simulink model "demo_comp_imu"  (R2025a)
settings: Solver=VariableStepAuto  StartTime=0.0  StopTime=5  RelTol=1e-3
settings Model: Creator=xing2  LastModifiedBy=xing2

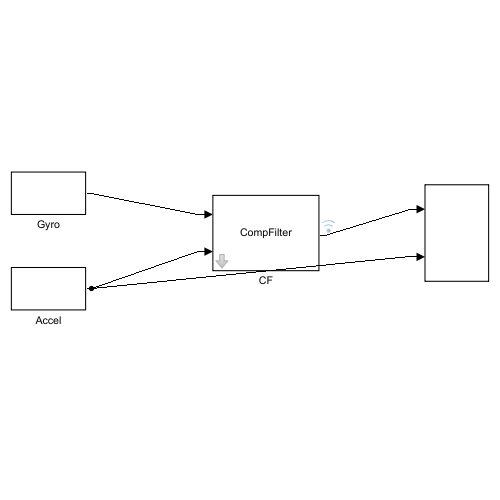
[thumbnail: Simulink's stored preview of the top-level diagram]
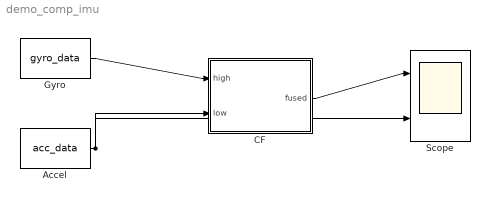
== system demo_comp_imu ==
  Accel : FromWorkspace  VariableName=acc_data
  CF : Subsystem  mask{alpha=0.98}
      mask prompts: alpha "alpha (0~1)"
      mask help: Complementary Filter: alpha*high + (1-alpha)*low
      mask Display: disp('CompFilter');
  Gyro : FromWorkspace  VariableName=gyro_data
  Scope : Scope  NumInputPorts=2
  wires:
  Gyro/1 -> CF/1(high)
  Accel/1 -> CF/2(low), Scope/2
  CF/1(fused) -> Scope/1

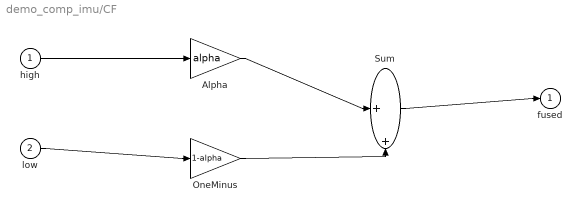
== system demo_comp_imu/CF ==
  high : Inport
  low : Inport  Port=2
  Alpha : Gain  Gain=alpha
  OneMinus : Gain  Gain=1-alpha
  Sum : Sum  Inputs=|++
  fused : Outport
  wires:
  Sum/1 -> fused/1
  OneMinus/1 -> Sum/2
  Alpha/1 -> Sum/1
  low/1 -> OneMinus/1
  high/1 -> Alpha/1
